simulink model "pir_based_control_pmsm_motors"  (R2024b)
settings: Solver=ode3  StartTime=0.0  StopTime=10.0  FixedStep=1e-7  RelTol=1e-3
undefined symbols (not defined in the file or in its folder): Ion, Lithium
libraries: spsIGBTDiodeLib x8, spsSeriesRLCBranchLib x4, spsBatteryLib x1, spsGroundLib x1, spsPermanentMagnetSynchronousMachineLib x1, spsThreePhaseVIMeasurementLib x1, spsVoltageMeasurementLib x1, sps_lib x1
settings Model: Creator=ravit  LastModifiedBy=ravit

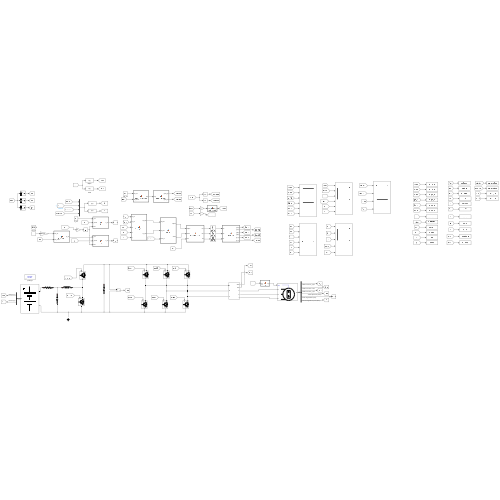
[thumbnail: Simulink's stored preview of the top-level diagram]
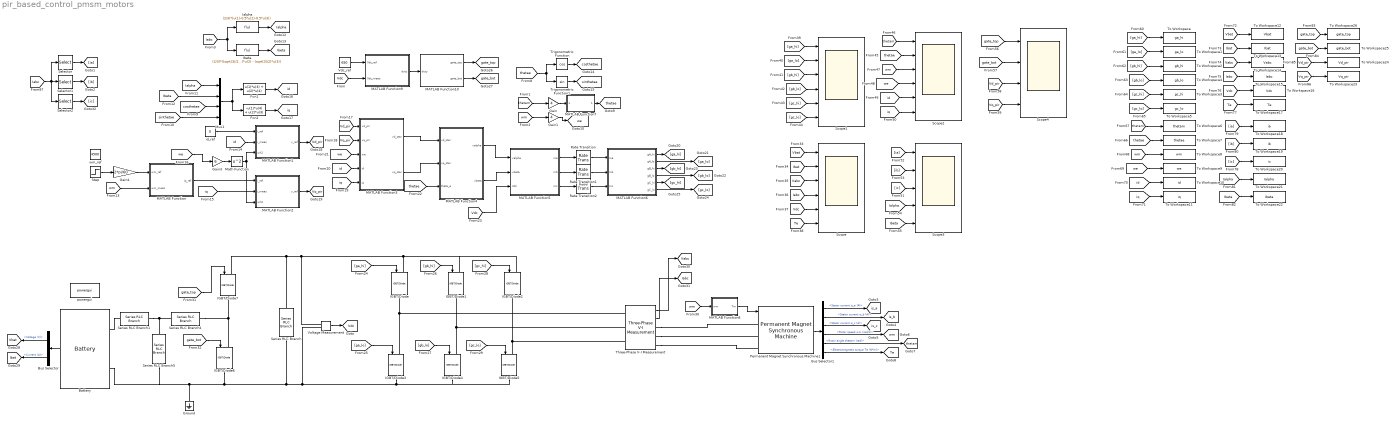
== system pir_based_control_pmsm_motors ==
  Battery : spsBatteryLib/Battery  BatType=Lithium-Ion  NomV=350  NomQ=150  SOC=80  Batt_Tr=10  PresetModel=on  MaxQ=150  MinV=262.5  FullV=407.3955  Dis_rate=65.2174  R=0.023333  Normal_OP=135.6522  expZone="[378.135      7.369565]"
  Bus Selector : BusSelector  OutputSignals=Voltage (V),Current (A)
  Bus Selector1 : BusSelector  OutputSignals=Stator current is_a (A),Stator current is_b (A),Stator current is_c (A),Rotor speed wm (rad/s),Rotor angle thetam (rad),Electromagnetic torque Te (N*m)
  Fcn1 : Fcn  Expr=u(1)*u(3) + u(2)*u(4)
  Fcn2 : Fcn  Expr=-u(1)*u(4) + u(2)*u(3)
  Gain : Gain  Gain=4
  Gain1 : Gain  Gain=4
  Gain3 : Gain  Gain=6
  Gain4 : Gain  Gain=2*pi/60
  Ground : spsGroundLib/Ground  LConnTagsString=a
  IGBT/Diode{,1..7} (8 alike) : spsIGBTDiodeLib/IGBT//Diode  Ron=1e-3  Rs=1e5  Cs=inf  Measurements=off
  Ialpha : Fcn  Expr=(2/3)*(u(1)-0.5*u(2)-0.5*u(3))
  Ibeta : Fcn  Expr=(2/3)*((sqrt(3)/2)*u(2) - (sqrt(3)/2)*u(3))
  MATLAB Function : MATLAB Function  TreatAsAtomicUnit=on
  MATLAB Function1 : MATLAB Function  TreatAsAtomicUnit=on
  MATLAB Function10 : MATLAB Function  TreatAsAtomicUnit=on
  MATLAB Function2 : MATLAB Function  TreatAsAtomicUnit=on
  MATLAB Function3 : MATLAB Function  TreatAsAtomicUnit=on
  MATLAB Function4 : MATLAB Function  TreatAsAtomicUnit=on
  MATLAB Function5 : MATLAB Function  TreatAsAtomicUnit=on
  MATLAB Function6 : MATLAB Function  TreatAsAtomicUnit=on
  MATLAB Function7 : MATLAB Function  TreatAsAtomicUnit=on
  MATLAB Function8 : MATLAB Function  TreatAsAtomicUnit=on
  MATLAB Function9 : MATLAB Function  TreatAsAtomicUnit=on
  Math Function : Math  Operator=square
  Mux1 : Mux
  Permanent Magnet Synchronous Machine1 : spsPermanentMagnetSynchronousMachineLib/Permanent Magnet Synchronous Machine  NbPhases=3  FluxDistribution=Sinusoidal  RotorType=Salient-pole  MechanicalLoad=Torque Tm  PresetModel=No  ShowDetailedParameters=on  MeasurementBus=off  Resistance=0.05  Inductance=8.5e-3  dqInductances=[0.20e-3, 0.30e-3]  La=0.000395  MachineConstant=Flux linkage established by magnets (V.s)  Flux=0.09  VoltageCst=65.2968  TorqueCst=0.54  Flat=120  Mechanical=[0.03, 0.008, 4, 0]  PolePairs=4  InitialConditions=[0,0, 0,0]  InitialConditions5ph=[0 0 0 0 0 0]  RefAngle=90 degrees behind phase A axis (modified Park)  IterativeDiscreteModel=Trapezoidal non iterative  TsBlock=-1  TsPowergui=0
  Rate Transition : RateTransition
  Rate Transition1 : RateTransition
  Rate Transition2 : RateTransition
  Scope : Scope  NumInputPorts=6
  Scope1 : Scope  NumInputPorts=6
  Scope2 : Scope  NumInputPorts=6
  Scope3 : Scope  NumInputPorts=5
  Scope4 : Scope  NumInputPorts=4
  Selector : Selector  InputPortWidth=3  IndexOptions=Index vector (dialog)  Indices=[1]  OutputSizes=1
  Selector1 : Selector  InputPortWidth=3  IndexOptions=Index vector (dialog)  Indices=[2]  OutputSizes=1
  Selector2 : Selector  InputPortWidth=3  IndexOptions=Index vector (dialog)  Indices=[3]  OutputSizes=1
  Series RLC Branch : spsSeriesRLCBranchLib/Series RLC Branch  LConnTagsString=__new0  RConnTagsString=__new0  BranchType=C  Resistance=1  Inductance=1e-3  SetiL0=off  InitialCurrent=0  Capacitance=500e-6  Setx0=on  InitialVoltage=900  Measurements=None
  Series RLC Branch1 : spsSeriesRLCBranchLib/Series RLC Branch  LConnTagsString=__new0  RConnTagsString=__new0  BranchType=R  Resistance=0.1  Inductance=190e-3  SetiL0=off  InitialCurrent=0  Capacitance=1e-6  Setx0=off  InitialVoltage=0  Measurements=None
  Series RLC Branch4 : spsSeriesRLCBranchLib/Series RLC Branch  LConnTagsString=__new0  RConnTagsString=__new0  BranchType=L  Resistance=0.1  Inductance=190e-3  SetiL0=off  InitialCurrent=0  Capacitance=1e-6  Setx0=off  InitialVoltage=0  Measurements=None
  Series RLC Branch5 : spsSeriesRLCBranchLib/Series RLC Branch  LConnTagsString=__new0  RConnTagsString=__new0  BranchType=C  Resistance=1  Inductance=1e-3  SetiL0=off  InitialCurrent=0  Capacitance=200e-6  Setx0=on  InitialVoltage=350  Measurements=None
  Step : Step  Time=5  After=4500  SampleTime=0
  Three-Phase V-I Measurement : spsThreePhaseVIMeasurementLib/Three-Phase V-I Measurement  VoltageMeasurement=phase-to-ground  SetLabelV=off  LabelV=Vabc  Vpu=off  VpuLL=off  CurrentMeasurement=yes  SetLabelI=off  LabelI=Iabc  Ipu=off  Pbase=100e6  Vbase=500e3  OutputType=Complex  PhasorSimulation=off  PSBequivalent=0
  To Workspace : ToWorkspace  VariableName=ga_hi  SaveFormat=Timeseries  SampleTime=-1
  To Workspace1 : ToWorkspace  VariableName=ga_lo  SaveFormat=Timeseries  SampleTime=-1
  To Workspace10 : ToWorkspace  VariableName=id  SaveFormat=Timeseries  SampleTime=-1
  To Workspace11 : ToWorkspace  VariableName=iq  SaveFormat=Timeseries  SampleTime=-1
  To Workspace12 : ToWorkspace  VariableName=Vbat  SaveFormat=Timeseries  SampleTime=-1
  To Workspace13 : ToWorkspace  VariableName=Ibat  SaveFormat=Timeseries  SampleTime=-1
  To Workspace14 : ToWorkspace  VariableName=Vabc  SaveFormat=Timeseries  SampleTime=-1
  To Workspace15 : ToWorkspace  VariableName=Iabc  SaveFormat=Timeseries  SampleTime=-1
  To Workspace16 : ToWorkspace  VariableName=Vdc  SaveFormat=Timeseries  SampleTime=-1
  To Workspace17 : ToWorkspace  VariableName=Te  SaveFormat=Timeseries  SampleTime=-1
  To Workspace18 : ToWorkspace  VariableName=ia  SaveFormat=Timeseries  SampleTime=-1
  To Workspace19 : ToWorkspace  VariableName=ib  SaveFormat=Timeseries  SampleTime=-1
  To Workspace2 : ToWorkspace  VariableName=gb_hi  SaveFormat=Timeseries  SampleTime=-1
  To Workspace20 : ToWorkspace  VariableName=ic  SaveFormat=Timeseries  SampleTime=-1
  To Workspace21 : ToWorkspace  VariableName=Ialpha  SaveFormat=Timeseries  SampleTime=-1
  To Workspace22 : ToWorkspace  VariableName=Ibeta  SaveFormat=Timeseries  SampleTime=-1
  To Workspace23 : ToWorkspace  VariableName=Vq_pir  SaveFormat=Timeseries  SampleTime=-1
  To Workspace24 : ToWorkspace  VariableName=Vd_pir  SaveFormat=Timeseries  SampleTime=-1
  To Workspace25 : ToWorkspace  VariableName=gate_bot  SaveFormat=Timeseries  SampleTime=-1
  To Workspace26 : ToWorkspace  VariableName=gate_top  SaveFormat=Timeseries  SampleTime=-1
  To Workspace3 : ToWorkspace  VariableName=gc_hi  SaveFormat=Timeseries  SampleTime=-1
  To Workspace4 : ToWorkspace  VariableName=gb_lo  SaveFormat=Timeseries  SampleTime=-1
  To Workspace5 : ToWorkspace  VariableName=gc_lo  SaveFormat=Timeseries  SampleTime=-1
  To Workspace6 : ToWorkspace  VariableName=thetam  SaveFormat=Timeseries  SampleTime=-1
  To Workspace7 : ToWorkspace  VariableName=thetae  SaveFormat=Timeseries  SampleTime=-1
  To Workspace8 : ToWorkspace  VariableName=wm  SaveFormat=Timeseries  SampleTime=-1
  To Workspace9 : ToWorkspace  VariableName=we  SaveFormat=Timeseries  SampleTime=-1
  Trigonometric Function : Trigonometry  Operator=cos
  Trigonometric Function1 : Trigonometry
  Vdc_ref : Constant  Value=650
  Voltage Measurement : spsVoltageMeasurementLib/Voltage Measurement  PhasorSimulation=off  OutputType=Complex  PSBequivalent=0
  id_ref : Constant  Value=0
  powergui : sps_lib/powergui  Priority=1  SimulationMode=Discrete  SampleTime=5e-6  frequency=60  Iterations=50  frequencyindice=0  Pbase=100e6  ErrMax=1e-4  UnitsV=kV  UnitsW=MW  buscounter=0  FunctionMessages=off  echomessages=off  EnableUseOfTLC=off  CurrentSourceSwitches=off  DisableSnubberDevices=off  DisableRonSwitches=off  DisableVfSwitches=off  DisplayEquations=off  AutomaticDiscreteSolvers=off  SolverType=Tustin/Backward Euler (TBE)  Interpol=off  ExternalGateDelay=off  methode=off  Ts=100  x0status=blocks  SPID=on  SwTol=0  HookPort=off  NonlinearTolerance=1e-4  nMaxIteration=100  ContinueOnMaxIteration=off  RestoreLinks=warning  ResistiveCurrentMeasurement=off  Frange=[0:2:500]  Ylog=off  Xlog=on  ShowGrid=off  save=off  variable=ZData  structure=0  ZoomFFT=off  StartTime=0.0  cycles=1  DisplayStyle=1  fundamental=60  FreqAxis=off  MaxFrequency=1000  frequencyindicesteady=1  RmsSteady=1  display=off
  wm_ref : Constant  Value=4500
  tag scope: Iabc=global, Ialpha=global, Ibat=global, Ibeta=global, Te=global, Vabc=global, Vbat=global, Vd_pir=global, Vdc=global, Vq_pir=global, costhetae=global, gate_bot=global, gate_top=global, id=global, iq=global, is_a=global, is_b=global, is_c=global, sinthetae=global, thetae=global, thetam=global, we=global, wm=global
  wires:
  Voltage Measurement/1 -> [Vdc]
  Battery/1 -> Bus Selector/1
  Permanent Magnet Synchronous Machine1/1 -> Bus Selector1/1
  Bus Selector1/1 -> [is_a]  "<Stator current is_a (A)>"
  Bus Selector1/2 -> [is_b]  "<Stator current is_b (A)>"
  Bus Selector1/3 -> [is_c]  "<Stator current is_c (A)>"
  Bus Selector1/4 -> [wm]  "<Rotor speed wm (rad/s)>"
  Bus Selector1/5 -> [thetam]  "<Rotor angle thetam (rad)>"
  Bus Selector1/6 -> [Te]  "<Electromagnetic torque Te (N*m)>"
  Gain/1 -> MATLAB Function7/1(theta_e_raw)
  [thetam] -> Gain/1
  MATLAB Function7/1(theta_e) -> [thetae]
  [wm] -> Gain1/1
  Gain1/1 -> [we]
  Ialpha/1 -> [Ialpha]
  Ibeta/1 -> [Ibeta]
  [thetae] -> Trigonometric Function/1, Trigonometric Function1/1
  Trigonometric Function/1 -> [costhetae]
  Trigonometric Function1/1 -> [sinthetae]
  [Ialpha] -> Mux1/1
  [Ibeta] -> Mux1/2
  [costhetae] -> Mux1/3
  [sinthetae] -> Mux1/4
  Mux1/1 -> Fcn1/1, Fcn2/1
  Fcn1/1 -> [id]
  Fcn2/1 -> [iq]
  [wm] -> MATLAB Function/2(wm_meas)
  [id] -> MATLAB Function1/2(i_meas)
  [we] -> Gain3/1
  Gain3/1 -> Math Function/1
  Math Function/1 -> MATLAB Function2/3(wh2), MATLAB Function1/3(wh2)
  [iq] -> MATLAB Function2/2(i_meas)
  id_ref/1 -> MATLAB Function1/1(i_ref)
  MATLAB Function/1(iq_ref) -> MATLAB Function2/1(i_ref)
  Gain4/1 -> MATLAB Function/1(wm_ref)
  MATLAB Function1/1(v_ref) -> [Vd_pir]
  MATLAB Function2/1(v_ref) -> [Vq_pir]
  [Vd_pir] -> MATLAB Function3/1(vd_pir)
  [Vq_pir] -> MATLAB Function3/2(vq_pir)
  [iq] -> MATLAB Function3/5(iq)
  [id] -> MATLAB Function3/4(id)
  [we] -> MATLAB Function3/3(we)
  MATLAB Function3/1(vd_star) -> MATLAB Function4/1(vd_star)
  MATLAB Function3/2(vq_star) -> MATLAB Function4/2(vq_star)
  [thetae] -> MATLAB Function4/3(theta_e)
  MATLAB Function4/1(valpha) -> MATLAB Function5/1(valpha)
  MATLAB Function4/2(vbeta) -> MATLAB Function5/2(vbeta)
  [Vdc] -> MATLAB Function5/3(Vdc)
  MATLAB Function5/1(ma) -> Rate Transition/1
  MATLAB Function5/2(mb) -> Rate Transition1/1
  MATLAB Function5/3(mc) -> Rate Transition2/1
  MATLAB Function6/1(gA_hi) -> [ga_hi]
  MATLAB Function6/2(gA_lo) -> [ga_lo]
  MATLAB Function6/4(gB_lo) -> [gb_lo]
  MATLAB Function6/3(gB_hi) -> [gb_hi]
  MATLAB Function6/6(gC_lo) -> [gc_lo]
  MATLAB Function6/5(gC_hi) -> [gc_hi]
  [ga_hi] -> IGBT/Diode/1
  [ga_lo] -> IGBT/Diode3/1
  [gb_hi] -> IGBT/Diode1/1
  [gb_lo] -> IGBT/Diode4/1
  [gc_hi] -> IGBT/Diode2/1
  [gc_lo] -> IGBT/Diode5/1
  Rate Transition/1 -> MATLAB Function6/1(ma)
  Rate Transition1/1 -> MATLAB Function6/2(mb)
  Rate Transition2/1 -> MATLAB Function6/3(mc)
  MATLAB Function8/1(Tm) -> Permanent Magnet Synchronous Machine1/1
  [wm] -> MATLAB Function8/1(wm)
  Vdc_ref/1 -> MATLAB Function9/1(Vdc_ref)
  [Vdc] -> MATLAB Function9/2(Vdc_meas)
  MATLAB Function9/1(duty) -> MATLAB Function10/1(duty)
  MATLAB Function10/1(gate_top) -> [gate_top]
  MATLAB Function10/2(gate_bot) -> [gate_bot]
  [gate_top] -> IGBT/Diode7/1
  [gate_bot] -> IGBT/Diode6/1
  Step/1 -> Gain4/1
  Bus Selector/1 -> [Vbat]  "<Voltage (V)>"
  Bus Selector/2 -> [Ibat]  "<Current (A)>"
  Three-Phase V-I Measurement/1 -> [Vabc]
  Three-Phase V-I Measurement/2 -> [Iabc]
  [Vbat] -> Scope/1
  [Ibat] -> Scope/2
  [Vabc] -> Scope/3
  [Iabc] -> Scope/4
  [Vdc] -> Scope/5
  [Te] -> Scope/6
  [ga_hi] -> Scope1/1
  [ga_lo] -> Scope1/2
  [gb_hi] -> Scope1/3
  [gb_lo] -> Scope1/4
  [gc_hi] -> Scope1/5
  [gc_lo] -> Scope1/6
  [thetam] -> Scope2/1
  [thetae] -> Scope2/2
  [wm] -> Scope2/3
  [we] -> Scope2/4
  [iq] -> Scope2/6
  [id] -> Scope2/5
  [ib] -> Scope3/2
  [ia] -> Scope3/1
  [ic] -> Scope3/3
  [Ibeta] -> Scope3/5
  [Ialpha] -> Scope3/4
  [Vq_pir] -> Scope4/4
  [Vd_pir] -> Scope4/3
  [gate_bot] -> Scope4/2
  [gate_top] -> Scope4/1
  [ga_hi] -> To Workspace/1
  [ga_lo] -> To Workspace1/1
  [gb_hi] -> To Workspace2/1
  [gc_hi] -> To Workspace3/1
  [gb_lo] -> To Workspace4/1
  [gc_lo] -> To Workspace5/1
  [thetam] -> To Workspace6/1
  [thetae] -> To Workspace7/1
  [wm] -> To Workspace8/1
  [we] -> To Workspace9/1
  [id] -> To Workspace10/1
  [iq] -> To Workspace11/1
  [Vbat] -> To Workspace12/1
  [Ibat] -> To Workspace13/1
  [Vabc] -> To Workspace14/1
  [Iabc] -> To Workspace15/1
  [Vdc] -> To Workspace16/1
  [Te] -> To Workspace17/1
  [ia] -> To Workspace18/1
  [ib] -> To Workspace19/1
  [ic] -> To Workspace20/1
  [Ialpha] -> To Workspace21/1
  [Ibeta] -> To Workspace22/1
  [Vq_pir] -> To Workspace23/1
  [Vd_pir] -> To Workspace24/1
  [gate_bot] -> To Workspace25/1
  [gate_top] -> To Workspace26/1
  [Iabc] -> Selector/1, Selector2/1, Selector1/1
  Selector/1 -> [ia]
  Selector1/1 -> [ib]
  Selector2/1 -> [ic]
  [Iabc] -> Ialpha/1, Ibeta/1
  connections:
  IGBT/Diode6/LConn1 -- Series RLC Branch4/RConn1 -- IGBT/Diode7/RConn1
  Voltage Measurement/LConn2 -- IGBT/Diode4/RConn1 -- IGBT/Diode5/RConn1 -- IGBT/Diode3/RConn1 -- Series RLC Branch/RConn1 -- Battery/LConn2 -- Series RLC Branch5/RConn1 -- Ground/LConn1 -- IGBT/Diode6/RConn1
  IGBT/Diode3/LConn1 -- IGBT/Diode/RConn1 -- Three-Phase V-I Measurement/LConn1
  IGBT/Diode4/LConn1 -- IGBT/Diode1/RConn1 -- Three-Phase V-I Measurement/LConn2
  IGBT/Diode5/LConn1 -- Three-Phase V-I Measurement/LConn3 -- IGBT/Diode2/RConn1
  Three-Phase V-I Measurement/RConn2 -- Permanent Magnet Synchronous Machine1/LConn2
  Three-Phase V-I Measurement/RConn1 -- Permanent Magnet Synchronous Machine1/LConn1
  Three-Phase V-I Measurement/RConn3 -- Permanent Magnet Synchronous Machine1/LConn3
  IGBT/Diode/LConn1 -- Voltage Measurement/LConn1 -- IGBT/Diode7/LConn1 -- Series RLC Branch/LConn1 -- IGBT/Diode2/LConn1 -- IGBT/Diode1/LConn1
  Battery/LConn1 -- Series RLC Branch1/LConn1
  Series RLC Branch1/RConn1 -- Series RLC Branch5/LConn1 -- Series RLC Branch4/LConn1

== matlab function pir_based_control_pmsm_motors/MATLAB Function9 ==
  data: Vdc_ref input; duty output; Vdc_meas input
function duty = DCDC_VoltageLoop(Vdc_ref, Vdc_meas)
% Outer voltage loop for bidirectional boost/buck converter
% Positive error (Vdc low) -> increase duty -> more boost action
% Negative error (Vdc high, e.g. regen dumping energy back) -> decrease
% duty -> converter allows buck path to remove energy from DC link

persistent int_state
if isempty(int_state)
    int_state = 0.46;   % pre-load near nominal duty (Vin=350V, Vout=650V => D=1-350/650=0.46)
end

% ---- Parameters ----
Kp = 0.002;      % proportional gain (duty per volt of error)
Ki = 0.05;       % integral gain
Ts = 5e-6;       % must match block sample time
D_max = 0.9;     % avoid D=1 (loses control authority / shoot-through risk)
D_min = 0.1;     % avoid D=0 (same reason, mirrored)

% ---- Error ----
e = Vdc_ref - Vdc_meas;

% ---- Proportional term ----
P_term = Kp * e;

% ---- Tentative integral update ----
int_tentative = int_state + Ki * e * Ts;

% ---- Unsaturated duty ----
d_unsat = P_term + int_tentative;

% ---- Saturate ----
duty = min(max(d_unsat, D_min), D_max);

% ---- Anti-windup: only commit integral if not saturating ----
if (d_unsat == duty)
    int_state = int_tentative;
end

end

== matlab function pir_based_control_pmsm_motors/MATLAB Function10 ==
  data: duty input; gate_top output; gate_bot output
function [gate_top, gate_bot] = DCDC_GateGen(duty)
% Sawtooth-carrier PWM with dead-time for bidirectional 2-switch
% boost/buck converter leg.
% Convention: gate_bot ON (duty fraction) = boost/charging inductor path
%             gate_top ON (1-duty fraction) = buck/regen path
% Complementary switching with dead-time between transitions.

persistent carrier
persistent prev_cmd
persistent delay_top delay_bot

if isempty(carrier)
    carrier = 0;
    prev_cmd = 0;
    delay_top = 0;
    delay_bot = 0;
end

% ---- Parameters ----
Ts_pwm = 1e-7;      % must match block sample time
fsw    = 10000;      % Hz, converter switching frequency
Tsw    = 1/fsw;
carrier_step = 1/round(Tsw/Ts_pwm);   % sawtooth 0->1, wraps every Tsw

dead_time = 1e-6;                     % seconds
dead_samples = round(dead_time/Ts_pwm);

% ---- Update sawtooth carrier (0 to 1, resets) ----
carrier = carrier + carrier_step;
if carrier >= 1
    carrier = carrier - 1;
end

% ---- Raw command: bottom switch ON when duty > carrier ----
cmd = double(duty >= carrier);

% ---- Dead-time state machine (bottom switch = "cmd", top = complementary) ----
if cmd == 1 && prev_cmd == 0
    delay_bot = dead_samples;
    delay_top = 0;
elseif cmd == 0 && prev_cmd == 1
    delay_top = dead_samples;
    delay_bot = 0;
end

cmd_bot_raw = cmd;
cmd_top_raw = double(~cmd);

if delay_bot > 0
    gate_bot = 0;
    delay_bot = delay_bot - 1;
else
    gate_bot = cmd_bot_raw;
end

if delay_top > 0
    gate_top = 0;
    delay_top = delay_top - 1;
else
    gate_top = cmd_top_raw;
end

prev_cmd = cmd;

end

== matlab function pir_based_control_pmsm_motors/MATLAB Function1 ==
  data: i_ref input; v_ref output; i_meas input; wh2 input
function v_ref = PIR_d(i_ref, i_meas, wh2)
% PIR current controller: PI (with anti-windup) + resonant term (biquad)

persistent int_ki e1 e2 y1 y2
if isempty(int_ki)
    int_ki = 0;
    e1 = 0; e2 = 0;
    y1 = 0; y2 = 0;
end

% ---- Parameters ----
Kp = 1.257;      % d-axis: 1.257 | q-axis: 1.885
Ki = 188.5;
wc = 62.8;
Kr = 80;
Ts = 5e-6;
V_max = 400;     % V, output saturation -- tune to your actual Vdc/2 or similar
V_min = -400;

% ---- Error ----
e = i_ref - i_meas;

% ---- Proportional ----
P_term = Kp * e;

% ---- Tentative integral update ----
int_tentative = int_ki + Ki * e * Ts;

% ---- Resonant term (bilinear biquad, unchanged from before) ----
wh = sqrt(max(wh2, 0));
c = 2/Ts;
a0 = c^2 + 2*wc*c + wh^2;
b0 =  2*Kr*wc*c / a0;
b2 = -2*Kr*wc*c / a0;
a1 = (2*wh^2 - 2*c^2) / a0;
a2 = (c^2 - 2*wc*c + wh^2) / a0;
y = b0*e + b2*e2 - a1*y1 - a2*y2;
R_term = y;

% ---- Unsaturated total output ----
v_unsat = P_term + int_tentative + R_term;

% ---- Saturate output ----
v_ref = min(max(v_unsat, V_min), V_max);

% ---- Anti-windup: only commit integral update if output not saturating ----
if (v_unsat == v_ref)
    int_ki = int_tentative;
end

% ---- Shift resonant filter delay states (always updates) ----
e2 = e1;
e1 = e;
y2 = y1;
y1 = y;

end

== matlab function pir_based_control_pmsm_motors/MATLAB Function ==
  data: wm_ref input; iq_ref output; wm_meas input
function iq_ref = Speed_PI(wm_ref, wm_meas)
% Discrete PI speed controller with anti-windup (clamping)
% Sample time Ts must match the block's discrete sample time setting

persistent int_state
if isempty(int_state)
    int_state = 0;
end

% ---- Parameters (tune here or promote to mask parameters) ----
Kp_w = 2;
Ki_w = 15;
Ts   = 5e-6;      % must match block sample time
i_max = 400;      % A, saturation / anti-windup limit
i_min = -400;

% ---- Error ----
werr = wm_ref - wm_meas;

% ---- Proportional term ----
P_term = Kp_w * werr;

% ---- Tentative integral update ----
int_tentative = int_state + Ki_w * werr * Ts;

% ---- Unsaturated output ----
u_unsat = P_term + int_tentative;

% ---- Saturate output ----
iq_ref = min(max(u_unsat, i_min), i_max);

% ---- Anti-windup: only commit integrator update if not saturating,
%      or if it would move the output back inside limits ----
if (u_unsat == iq_ref)
    int_state = int_tentative;   % no saturation, commit normally
end
% else: hold previous int_state (clamped) — this is the anti-windup action

end

== matlab function pir_based_control_pmsm_motors/MATLAB Function2 ==
  data: i_ref input; v_ref output; i_meas input; wh2 input
function v_ref = PIR_d(i_ref, i_meas, wh2)
% PIR current controller: PI (with anti-windup) + resonant term (biquad)

persistent int_ki e1 e2 y1 y2
if isempty(int_ki)
    int_ki = 0;
    e1 = 0; e2 = 0;
    y1 = 0; y2 = 0;
end

% ---- Parameters ----
Kp = 1.885;      % d-axis: 1.257 | q-axis: 1.885
Ki = 188.5;
wc = 62.8;
Kr = 80;
Ts = 5e-6;
V_max = 400;     % V, output saturation -- tune to your actual Vdc/2 or similar
V_min = -400;

% ---- Error ----
e = i_ref - i_meas;

% ---- Proportional ----
P_term = Kp * e;

% ---- Tentative integral update ----
int_tentative = int_ki + Ki * e * Ts;

% ---- Resonant term (bilinear biquad, unchanged from before) ----
wh = sqrt(max(wh2, 0));
c = 2/Ts;
a0 = c^2 + 2*wc*c + wh^2;
b0 =  2*Kr*wc*c / a0;
b2 = -2*Kr*wc*c / a0;
a1 = (2*wh^2 - 2*c^2) / a0;
a2 = (c^2 - 2*wc*c + wh^2) / a0;
y = b0*e + b2*e2 - a1*y1 - a2*y2;
R_term = y;

% ---- Unsaturated total output ----
v_unsat = P_term + int_tentative + R_term;

% ---- Saturate output ----
v_ref = min(max(v_unsat, V_min), V_max);

% ---- Anti-windup: only commit integral update if output not saturating ----
if (v_unsat == v_ref)
    int_ki = int_tentative;
end

% ---- Shift resonant filter delay states (always updates) ----
e2 = e1;
e1 = e;
y2 = y1;
y1 = y;

end

== matlab function pir_based_control_pmsm_motors/MATLAB Function3 ==
  data: vd_pir input; vd_star output; vq_pir input; we input; id input; iq input; vq_star output
function [vd_star, vq_star] = Decoupling(vd_pir, vq_pir, we, id, iq)
% Cross-coupling feedforward terms for IPMSM current control
% vd = ... - we*Lq*iq
% vq = ... + we*Ld*id + we*lambda_m

% ---- Motor parameters ----
Ld = 0.20e-3;      % H
Lq = 0.30e-3;      % H
lambda_m = 0.09;   % Wb

% ---- Feedforward terms ----
vd_ff = -we * Lq * iq;
vq_ff =  we * Ld * id + we * lambda_m;

% ---- Combine with PIR outputs ----
vd_star = vd_pir + vd_ff;
vq_star = vq_pir + vq_ff;

end

== matlab function pir_based_control_pmsm_motors/MATLAB Function4 ==
  data: vd_star input; valpha output; vq_star input; theta_e input; vbeta output
function [valpha, vbeta] = InvPark(vd_star, vq_star, theta_e)
% Inverse Park transform: dq -> alpha-beta
% valpha = vd*cos(theta_e) - vq*sin(theta_e)
% vbeta  = vd*sin(theta_e) + vq*cos(theta_e)

c = cos(theta_e);
s = sin(theta_e);

valpha = vd_star*c - vq_star*s;
vbeta  = vd_star*s + vq_star*c;

end

== matlab function pir_based_control_pmsm_motors/MATLAB Function5 ==
  data: valpha input; ma output; vbeta input; Vdc input; mb output; mc output
function [ma, mb, mc] = InvClarke_Norm(valpha, vbeta, Vdc)
% Inverse Clarke transform: alpha-beta -> abc, then normalize by Vdc
% va = valpha
% vb = -0.5*valpha + (sqrt(3)/2)*vbeta
% vc = -0.5*valpha - (sqrt(3)/2)*vbeta

va = valpha;
vb = -0.5*valpha + (sqrt(3)/2)*vbeta;
vc = -0.5*valpha - (sqrt(3)/2)*vbeta;

% ---- Protect against divide-by-zero / Vdc collapse ----
Vdc_min = 50;   % V, floor to avoid numerical blow-up if Vdc sags
Vdc_safe = max(Vdc, Vdc_min);

ma = va / Vdc_safe;
mb = vb / Vdc_safe;
mc = vc / Vdc_safe;

% ---- Clip to valid modulation range (avoids overmodulation for now) ----
ma = min(max(ma, -1), 1);
mb = min(max(mb, -1), 1);
mc = min(max(mc, -1), 1);

end

== matlab function pir_based_control_pmsm_motors/MATLAB Function6 ==
  data: ma input; gA_hi output; mb input; mc input; gA_lo output; gB_hi output; gB_lo output; gC_hi output; gC_lo output
function [gA_hi, gA_lo, gB_hi, gB_lo, gC_hi, gC_lo] = PWM_Gen(ma, mb, mc)
% Sine-triangle PWM with dead-time insertion
% Carrier: digitally generated triangle wave, -1 to +1
% Dead-time: delays each leg's turn-ON transition, turn-OFF is immediate

persistent carrier dir
persistent prevA prevB prevC
persistent delayA_hi delayA_lo delayB_hi delayB_lo delayC_hi delayC_lo

if isempty(carrier)
    carrier = -1;
    dir = 1;
    prevA = 0; prevB = 0; prevC = 0;
    delayA_hi = 0; delayA_lo = 0;
    delayB_hi = 0; delayB_lo = 0;
    delayC_hi = 0; delayC_lo = 0;
end

% ---- Parameters ----
Ts_pwm   = 1e-7;    % must match block sample time
fsw      = 10000;   % Hz
Tsw      = 1/fsw;
N_half   = round((Tsw/2)/Ts_pwm);   % samples per carrier half-period
carrier_step = 2/N_half;            % amplitude step per sample (span=2, -1 to 1)

dead_time = 1e-6;                   % seconds, IGBT dead-time
dead_samples = round(dead_time/Ts_pwm);

% ---- Update triangle carrier ----
carrier = carrier + dir*carrier_step;
if carrier >= 1
    carrier = 1;
    dir = -1;
elseif carrier <= -1
    carrier = -1;
    dir = 1;
end

% ---- Raw (ideal, no dead-time) switching command: 1 = upper ON ----
% Cast to double immediately -- comparisons return logical, which
% MATLAB Function code-gen will not allow mixing with double later.
cmdA = double(ma >= carrier);
cmdB = double(mb >= carrier);
cmdC = double(mc >= carrier);

% ---- Dead-time state machine per leg ----
[gA_hi, gA_lo, prevA, delayA_hi, delayA_lo] = ...
    apply_deadtime(cmdA, prevA, delayA_hi, delayA_lo, dead_samples);
[gB_hi, gB_lo, prevB, delayB_hi, delayB_lo] = ...
    apply_deadtime(cmdB, prevB, delayB_hi, delayB_lo, dead_samples);
[gC_hi, gC_lo, prevC, delayC_hi, delayC_lo] = ...
    apply_deadtime(cmdC, prevC, delayC_hi, delayC_lo, dead_samples);

end

% ---- Local function: dead-time logic for one leg ----
function [g_hi, g_lo, prev_cmd, d_hi, d_lo] = ...
         apply_deadtime(cmd, prev_cmd, d_hi, d_lo, dead_samples)

% All variables here are double throughout -- no logical anywhere
if cmd == 1 && prev_cmd == 0
    % Rising edge requested: start delay before turning hi ON
    d_hi = dead_samples;
    d_lo = 0;
elseif cmd == 0 && prev_cmd == 1
    % Falling edge requested: start delay before turning lo ON
    d_lo = dead_samples;
    d_hi = 0;
end

% Turn OFF immediately based on commanded state (double, not logical)
g_hi_raw = cmd;              % already double (0 or 1)
g_lo_raw = double(~cmd);     % cast the NOT result to double

% Count down delay; hold the "turning on" side LOW until delay elapses
if d_hi > 0
    g_hi = 0;
    d_hi = d_hi - 1;
else
    g_hi = g_hi_raw;
end

if d_lo > 0
    g_lo = 0;
    d_lo = d_lo - 1;
else
    g_lo = g_lo_raw;
end

prev_cmd = cmd;

end

== matlab function pir_based_control_pmsm_motors/MATLAB Function7 ==
  data: theta_e_raw input; theta_e output
function theta_e = Theta_e_Wrap(theta_e_raw)
% Wraps electrical angle to [0, 2*pi)
% mod() handles negative inputs correctly (unlike rem),
% which matters during speed reversal (we < 0)

theta_e = mod(theta_e_raw, 2*pi);

end

== matlab function pir_based_control_pmsm_motors/MATLAB Function8 ==
  data: wm input; Tm output
function Tm = Vehicle_Load(wm)
% Simplified road-load model converted to motor-shaft torque
% Flat road, constant-speed cruise approximation (no acceleration term
% here -- add dv/dt term if you want launch/acceleration transients)

% ---- Vehicle parameters (typical compact EV) ----
m    = 1500;      % kg, vehicle mass
g    = 9.81;      % m/s^2
Cr   = 0.012;     % rolling resistance coefficient
rho  = 1.225;     % kg/m^3, air density
Cd   = 0.29;      % drag coefficient
A    = 2.2;       % m^2, frontal area
Rw   = 0.30;      % m, wheel radius
Gr   = 9.0;       % gear ratio (motor to wheel)

% ---- Convert motor speed to vehicle speed ----
wwheel = wm / Gr;          % rad/s at wheel
v = wwheel * Rw;           % m/s, vehicle speed

% ---- Road load force ----
F_roll = m*g*Cr;
F_drag = 0.5*rho*Cd*A*v^2;
F_total = F_roll + F_drag;

% ---- Reflect to motor shaft ----
Tm = (F_total * Rw) / Gr;

end
